simulink model "asm1_test_ol"  (R2024a)
settings: Solver=ode15s  StartTime=0.0  StopTime=50  FixedStep=0.01  RelTol=1e-5  AbsTol=1e-8
values from neighbouring files (symbols this model uses):
  ACTIVATE = [ 0 ]    [init_bsm1.m]    (also in init_bsm2.m)
  carb3 = 0    [reginit_bsm1.m]    (also in reginit_bsm2.m)
  KLa3 = 240    [reginit_bsm1.m]    (also in reginit_bsm2.m = 120)
  TEMPMODEL = [ 0 ]    [init_bsm1.m]    (also in init_bsm2.m)
undefined symbols (not defined in the file or in its folder): PAR3, SOSAT3, VOL3, XINIT3
settings Model: Creator=ielulf  LastModifiedBy=Miederer
settings SolverCC: AutoScaleAbsTol=off  AlgebraicLoopSolver=TrustRegion
settings DataIOCC: InitialState=xFinal  SaveFormat=Array  SignalLoggingSaveFormat=ModelDataLogs  SaveOutput=off  ReturnWorkspaceOutputs=off  TimeSaveName=t  SignalLoggingName=sigsOut  OutputOption=SpecifiedOutputTimes  OutputTimes=[0:(1/96):50]
settings OptimizationCC: BlockReduction=off  BooleanDataType=off  OptimizeBlockIOStorage=off  BufferReuse=off  GlobalBufferReuse=off  ExpressionFolding=off  LocalBlockOutputs=off  InitFltsAndDblsToZero=on  LifeSpan=inf  OptimizeDataStoreBuffers=off  BusAssignmentInplaceUpdate=off
settings DebuggingCC: SaveWithParameterizedLinksMsg=none  UnderspecifiedInitializationDetection=Classic  MergeDetectMultiDrivingBlocksExec=none  SignalResolutionControl=TryResolveAllWithWarning  InheritedTsInSrcMsg=none  MultiTaskDSMMsg=warning  MultiTaskCondExecSysMsg=none  FcnCallInpInsideContextMsg=warning  UnconnectedInputMsg=warning  UnconnectedLineMsg=warning  SFUnexpectedBacktrackingDiag=warning  SFNoUnconditionalDefaultTransitionDiag=warning  SFExecutionAtInitializationDiag=none  ArithmeticOperatorsInVariantConditions=warning
settings HardwareCC: ProdBitPerPointer=32  ProdBitPerSizeT=32  ProdBitPerPtrDiffT=32  ProdLargestAtomicFloat=None  ProdIntDivRoundTo=Undefined  ProdEndianess=Unspecified  ProdWordSize=32  ProdHWDeviceType=32-bit Generic  TargetUnknown=on
settings ModelReferenceCC: EnableRefExpFcnMdlSchedulingChecks=on  PropagateSignalLabelsOutOfModel=off
settings RTWCC: TemplateMakefile=grt_unix.tmf  GPUComputeCapability=3.5  DLArmComputeVersion=19.05
settings CodeAppCC: StateflowObjectComments=on
settings GRTTargetCC: TargetFcnLib=ansi_tfl_tmw.mat  TargetLangStandard=C89/C90 (ANSI)  CombineOutputUpdateFcns=off  GRTInterface=on
settings ConfigComp: CovMetricSettings=dw  CovSaveCumulativeToWorkspaceVar=on  CovSaveSingleToWorkspaceVar=on

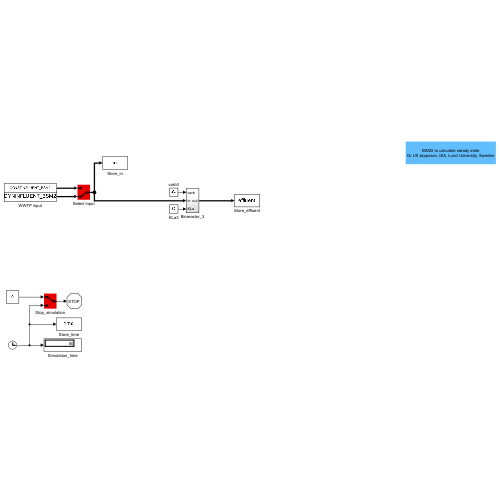
[thumbnail: Simulink's stored preview of the top-level diagram]
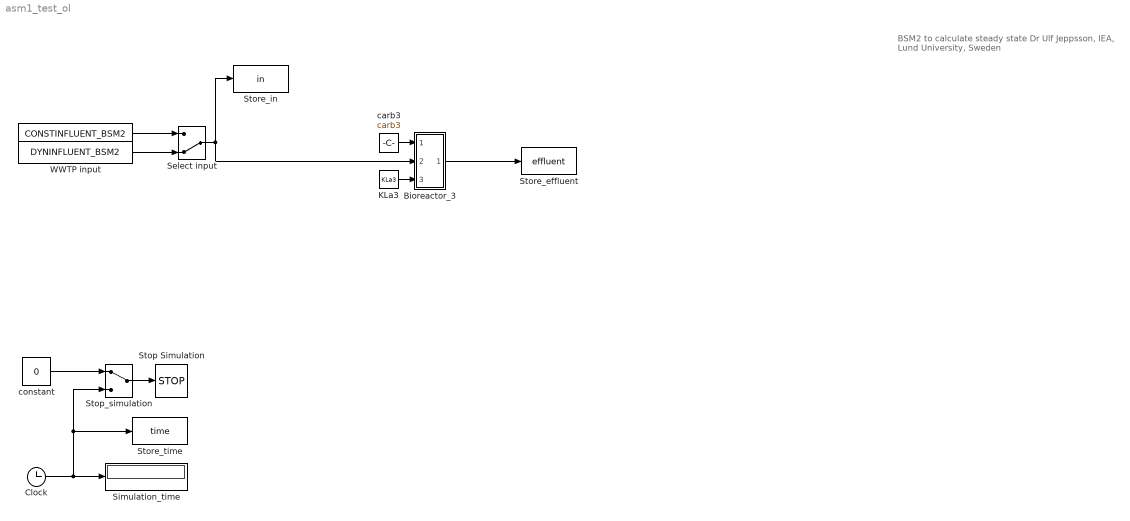
== system asm1_test_ol ==
  note: BSM2 to calculate steady state
      |  Dr Ulf Jeppsson, IEA, Lund University, Sweden
  " " : FromWorkspace  VariableName=CONSTINFLUENT_BSM2  SampleTime=-1  ZeroCross=off  OutputAfterFinalValue=Holding final value
  " constant" : Constant  Value=0
  Bioreactor_3 : Subsystem
  Clock : Clock
  KLa3 : Constant  Value=KLa3
  Select input : ManualSwitch  CurrentSetting=0
  Simulation_time : Display
  Stop Simulation : Stop
  Stop_simulation : ManualSwitch
  Store_effluent : ToWorkspace  VariableName=effluent
  Store_in : ToWorkspace  VariableName=in
  Store_time : ToWorkspace  VariableName=time
  WWTP input : FromWorkspace  VariableName=DYNINFLUENT_BSM2  SampleTime=-1  ZeroCross=off  OutputAfterFinalValue=Holding final value
  carb3 : Constant  Value=carb3
  wires:
  Clock/1 -> Simulation_time/1, Stop_simulation/2, Store_time/1
  Stop_simulation/1 -> Stop Simulation/1
  " constant"/1 -> Stop_simulation/1
  " "/1 -> Select input/1
  WWTP input/1 -> Select input/2
  carb3/1 -> Bioreactor_3/1(carb)
  KLa3/1 -> Bioreactor_3/3(KLa)
  Bioreactor_3/1(out) -> Store_effluent/1
  Select input/1 -> Bioreactor_3/2(in), Store_in/1

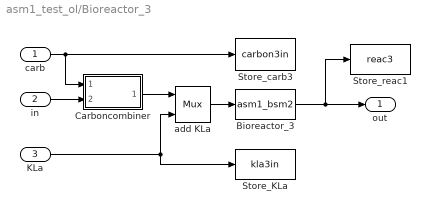
== system asm1_test_ol/Bioreactor_3 ==
  carb : Inport
  in : Inport  Port=2
  KLa : Inport  Port=3
  Bioreactor_3 : S-Function  FunctionName=asm1_bsm2  Parameters=XINIT3,PAR3,VOL3,SOSAT3,TEMPMODEL,ACTIVATE  SFunctionDeploymentMode=off  EnableBusSupport=off
  Carboncombiner : Subsystem
  Store_KLa : ToWorkspace  VariableName=kla3in  SampleTime=-1
  Store_carb3 : ToWorkspace  VariableName=carbon3in  SampleTime=-1
  Store_reac1 : ToWorkspace  VariableName=reac3  SampleTime=-1
  add KLa : Mux  Inputs=2
  out : Outport
  wires:
  KLa/1 -> Store_KLa/1, add KLa/2
  in/1 -> Carboncombiner/2(Input)
  carb/1 -> Store_carb3/1, Carboncombiner/1(C_flow)
  Carboncombiner/1(Output) -> add KLa/1
  add KLa/1 -> Bioreactor_3/1
  Bioreactor_3/1 -> Store_reac1/1, out/1

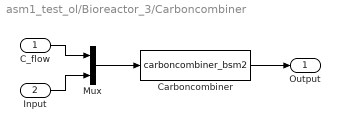
== system asm1_test_ol/Bioreactor_3/Carboncombiner ==
  C_flow : Inport
  Input : Inport  Port=2
  Carboncombiner : S-Function  FunctionName=carboncombiner_bsm2  Parameters=CARBONSOURCECONC  SFunctionDeploymentMode=off  EnableBusSupport=off
  Mux : Mux  Inputs=2
  Output : Outport
  wires:
  C_flow/1 -> Mux/1
  Mux/1 -> Carboncombiner/1
  Carboncombiner/1 -> Output/1
  Input/1 -> Mux/2
